simulink model "Example"  (R2021b)
settings: Solver=FixedStepDiscrete  StartTime=0.0  StopTime=10.0  FixedStep=1  RelTol=1e-3
settings Model: Creator=AAwdallah  LastModifiedBy=AAwdallah

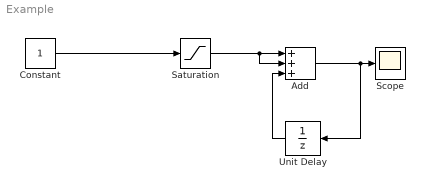
== system Example ==
  Add : Sum  Inputs=+++
  Constant : Constant
  Saturation : Saturate
  Scope : Scope
  Unit Delay : UnitDelay  SampleTime=-1  HasFrameUpgradeWarning=on
  wires:
  Constant/1 -> Saturation/1
  Saturation/1 -> Add/2, Add/1
  Add/1 -> Unit Delay/1, Scope/1
  Unit Delay/1 -> Add/3
